simulink model "FMHackTX"  (R2022b)
settings: Solver=VariableStepAuto  StartTime=0.0  StopTime=inf  RelTol=1e-3
model workspace (MAT data in the model file):
  SampleRate = 2000000
  f0 = 88900000
undefined symbols (not defined in the file): designMultirateFIR
libraries: dspsnks4 x1, dspmlti4 x1, commanabbnd3 x1, dspvision x1, hackrf_library x1
settings Model: Creator=gitud1  LastModifiedBy=gitud1

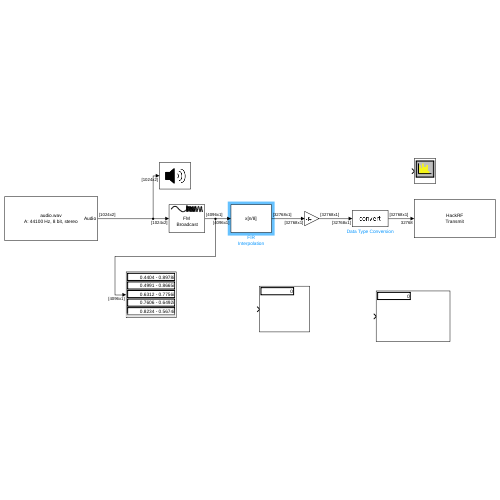
[thumbnail: Simulink's stored preview of the top-level diagram]
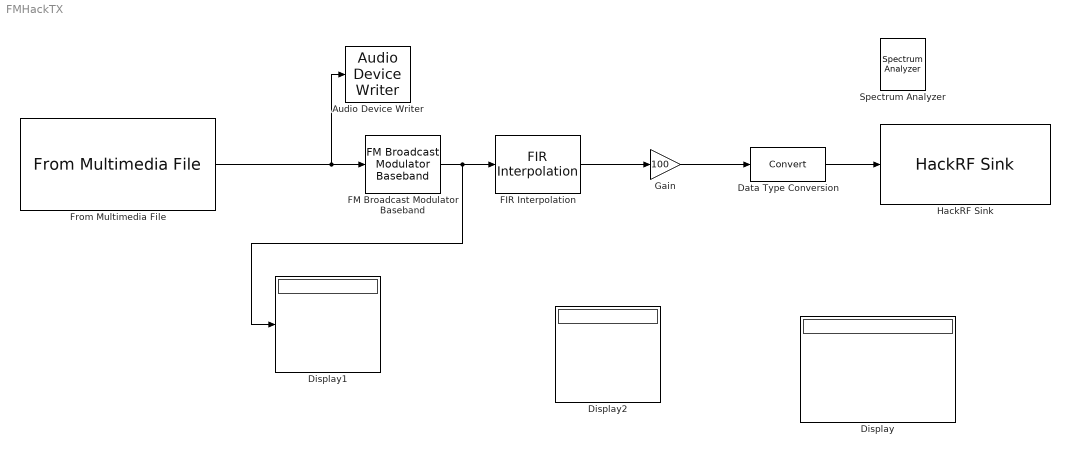
== system FMHackTX ==
  Audio Device Writer : dspsnks4/Audio Device Writer  Driver=ALSA  Device=Default  InheritSampleRate=on  SampleRate=44100  BitDepth=16-bit integer  BufferSize=4096  NumBuffers=10  DefaultOutputChannelMapping=on  OutputChannelMapping=1:2  OutputNumUnderrunSamples=off  DriverIdx=8  DeviceWarnFlag=''
  Data Type Conversion : DataTypeConversion  SaturateOnIntegerOverflow=off  RndMeth=Floor
  Display : Display
  Display1 : Display
  Display2 : Display
  FIR Interpolation : dspmlti4/FIR Interpolation  FilterSource=Auto  PrivateCoeffs=0  h=designMultirateFIR(3,1)  L=8  FilterObject=FINTERP  InputProcessing=Columns as channels (frame based)  framing=Enforce single-rate processing  outputBufInitCond=0  roundingMode=Floor  overflowMode=off  firstCoeffDataTypeStr=Inherit: Same word length as input  firstCoeffMin=[]  firstCoeffMax=[]  firstCoeffLastDataTypeStr=Inherit: Same word length as input  outputDataTypeStr=Inherit: Same as accumulator  outputMin=[]  outputMax=[]  outputLastDataTypeStr=Inherit: Same as accumulator
  FM Broadcast Modulator Baseband : commanabbnd3/FM Broadcast Modulator Baseband  SampleRate=192e3  FrequencyDeviation=75e3  FilterTimeConstant=75e-6  AudioSampleRate=48e3  Stereo=on  RBDS=off  RBDSSamplesPerSymbol=10  SimulateUsing=Code generation
  From Multimedia File : dspvision/From Multimedia File  inputFilename=/home/gitud1/Descargas/tesis/Pruebas/audio.wav  readRange=[1 Inf]  loop=on  numPlays=inf  outputStreams=Audio only  videoDataType=single  audioDataType=double  inheritSampleTime=on  userDefinedSampleTime=1/30  noAudioOutput=off  isIntensityVideo=off  fourcc=RGB  colorVideoFormat=One multidimensional signal  outputEOF=off  dataOrg=Column-major  audioFrameSize=1024  computeAudioFrameSize=off  outSamplingMode=Sample based
      settings: LibrarySourceBlock=visionsources/From Multimedia File
  Gain : Gain  Gain=100
  HackRF Sink : hackrf_library/HackRF Sink  hackrf_frequency=89.5e6  hackrf_bandwidth=1e6  hackrf_txvga=47.0
      settings: SourceProductName=HackRF
  Spectrum Analyzer : SpectrumAnalyzer
  wires:
  From Multimedia File/1 -> Audio Device Writer/1, FM Broadcast Modulator Baseband/1
  Data Type Conversion/1 -> HackRF Sink/1
  FM Broadcast Modulator Baseband/1 -> FIR Interpolation/1, Display1/1
  Gain/1 -> Data Type Conversion/1
  FIR Interpolation/1 -> Gain/1
